simulink model "UnifiedControlVehicleController"  (R2026b)
settings: Solver=FixedStepDiscrete  StopTime=0.1  FixedStep=UnifiedControlSampleTime
undefined symbols (not defined in the file): UnifiedControlMaximumAcceleration, UnifiedControlMaximumDeceleration, UnifiedControlVehicleMass
settings Model: DataDictionary=VehicleData.sldd  Creator=Xu Dingyi  LastModifiedBy=29358

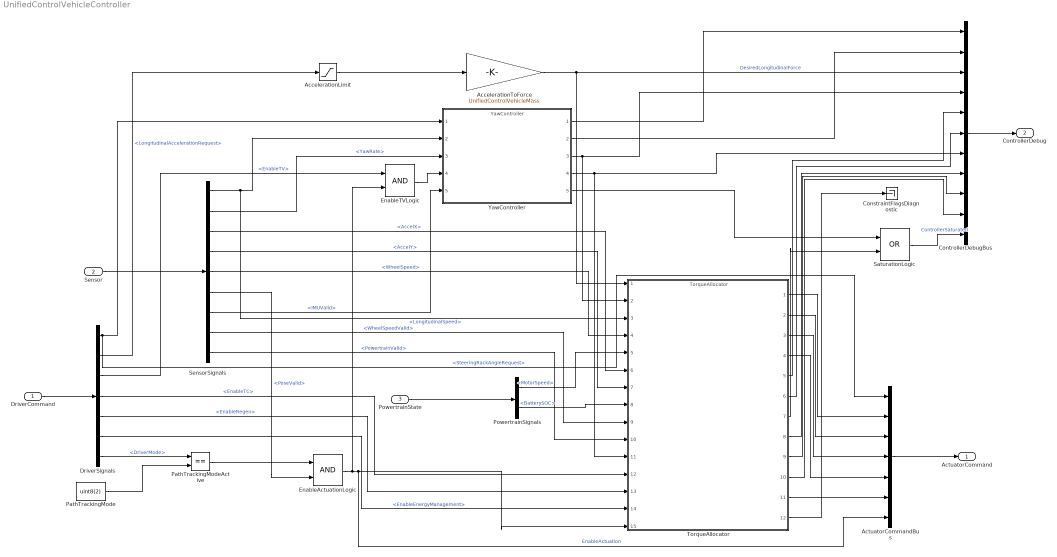
== system UnifiedControlVehicleController ==
  DriverCommand : Inport  OutDataTypeStr=Bus: DriverCommandBus
  Sensor : Inport  Port=2  OutDataTypeStr=Bus: SensorBus
  PowertrainState : Inport  Port=3  OutDataTypeStr=Bus: PowertrainStateBus
  AccelerationLimit : Saturate  UpperLimit=UnifiedControlMaximumAcceleration  LowerLimit=-UnifiedControlMaximumDeceleration
  AccelerationToForce : Gain  Gain=UnifiedControlVehicleMass
  ActuatorCommandBus : BusCreator  Inputs=7  OutDataTypeStr=Bus: ActuatorCommandBus
  ConstraintFlagsDiagnostic : Terminator
  ControllerDebugBus : BusCreator  Inputs=11  OutDataTypeStr=Bus: ControllerDebugBus
  DriverSignals : BusSelector  OutputSignals=SteeringRackAngleRequest,LongitudinalAccelerationRequest,EnableTV,EnableTC,EnableRegen,EnableEnergyManagement,DriverMode
  EnableActuationLogic : Logic  IconShape=distinctive
  EnableTVLogic : Logic  IconShape=distinctive
  PathTrackingMode : Constant  Value=uint8(2)  OutDataTypeStr=uint8
  PathTrackingModeActive : RelationalOperator  Operator===
  PowertrainSignals : BusSelector  OutputSignals=MotorSpeed,BatterySOC
  SaturationLogic : Logic  Operator=OR  IconShape=distinctive
  SensorSignals : BusSelector  OutputSignals=LongitudinalSpeed,YawRate,AccelX,AccelY,WheelSpeed,PoseValid,IMUValid,WheelSpeedValid,PowertrainValid
  TorqueAllocator : ModelReference  ModelNameDialog=TorqueAllocator  ModelReferenceVersion=2.0
  YawController : ModelReference  ModelNameDialog=YawController  ModelReferenceVersion=1.4
  ActuatorCommand : Outport  OutDataTypeStr=Bus: ActuatorCommandBus
  ControllerDebug : Outport  Port=2  OutDataTypeStr=Bus: ControllerDebugBus
  wires:
  DriverSignals/6 -> TorqueAllocator/14  "<EnableEnergyManagement>"
  DriverSignals/2 -> AccelerationLimit/1  "<LongitudinalAccelerationRequest>"
  YawController/2 -> ControllerDebugBus/2
  SensorSignals/9 -> TorqueAllocator/10  "<PowertrainValid>"
  DriverCommand/1 -> DriverSignals/1
  DriverSignals/4 -> TorqueAllocator/12  "<EnableTC>"
  YawController/4 -> ControllerDebugBus/7, TorqueAllocator/11
  Sensor/1 -> SensorSignals/1
  DriverSignals/5 -> TorqueAllocator/13  "<EnableRegen>"
  AccelerationLimit/1 -> AccelerationToForce/1
  DriverSignals/1 -> YawController/1, ActuatorCommandBus/1  "<SteeringRackAngleRequest>"
  DriverSignals/3 -> EnableTVLogic/1  "<EnableTV>"
  SensorSignals/6 -> EnableActuationLogic/2  "<PoseValid>"
  DriverSignals/7 -> PathTrackingModeActive/1  "<DriverMode>"
  PathTrackingMode/1 -> PathTrackingModeActive/2
  PathTrackingModeActive/1 -> EnableActuationLogic/1
  SensorSignals/1 -> TorqueAllocator/3, YawController/2  "<LongitudinalSpeed>"
  SensorSignals/2 -> YawController/3  "<YawRate>"
  SensorSignals/3 -> TorqueAllocator/6  "<AccelX>"
  SensorSignals/4 -> TorqueAllocator/7  "<AccelY>"
  EnableActuationLogic/1 -> TorqueAllocator/15, ActuatorCommandBus/7, EnableTVLogic/2  "EnableActuation"
  SensorSignals/5 -> TorqueAllocator/4  "<WheelSpeed>"
  SensorSignals/7 -> YawController/5  "<IMUValid>"
  YawController/1 -> ControllerDebugBus/1
  SensorSignals/8 -> TorqueAllocator/9  "<WheelSpeedValid>"
  EnableTVLogic/1 -> YawController/4
  PowertrainSignals/2 -> TorqueAllocator/8  "<BatterySOC>"
  PowertrainState/1 -> PowertrainSignals/1
  AccelerationToForce/1 -> ControllerDebugBus/3, TorqueAllocator/1  "DesiredLongitudinalForce"
  YawController/3 -> ControllerDebugBus/4, TorqueAllocator/2
  PowertrainSignals/1 -> TorqueAllocator/5  "<MotorSpeed>"
  YawController/5 -> SaturationLogic/1
  TorqueAllocator/1 -> ActuatorCommandBus/2
  TorqueAllocator/2 -> ActuatorCommandBus/3
  TorqueAllocator/3 -> ActuatorCommandBus/4
  TorqueAllocator/4 -> ActuatorCommandBus/5
  TorqueAllocator/5 -> ControllerDebugBus/5
  TorqueAllocator/6 -> ControllerDebugBus/6
  TorqueAllocator/7 -> SaturationLogic/2
  TorqueAllocator/8 -> ControllerDebugBus/8
  TorqueAllocator/9 -> ControllerDebugBus/9
  TorqueAllocator/10 -> ControllerDebugBus/10
  TorqueAllocator/11 -> ActuatorCommandBus/6
  TorqueAllocator/12 -> ConstraintFlagsDiagnostic/1
  SaturationLogic/1 -> ControllerDebugBus/11  "ControllerSaturated"
  ActuatorCommandBus/1 -> ActuatorCommand/1
  ControllerDebugBus/1 -> ControllerDebug/1
